simulink model "Bicycle_model_start"  (R2018a)
settings: Solver=VariableStepAuto  StartTime=0.0  StopTime=10.0  RelTol=1e-3
undefined symbols (not defined in the file): Ca, Cx, J, lf, lr, m, rwheel
libraries: simulink x1
settings Model: Creator=DvanHanswijk  LastModifiedBy=DvanHanswijk

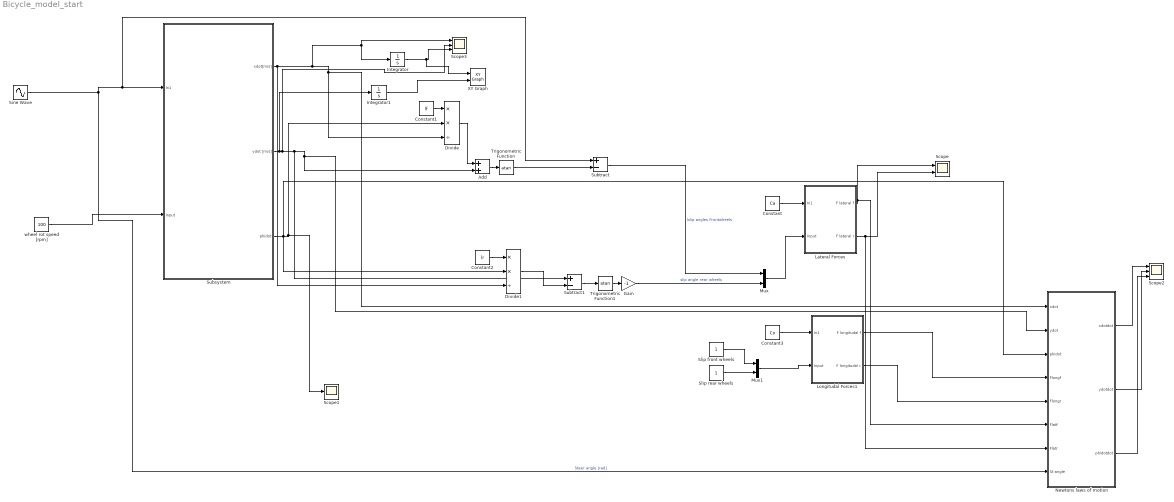
== system Bicycle_model_start ==
  Add : Sum
  Constant : Constant  Value=Ca
  Constant1 : Constant  Value=lf
  Constant2 : Constant  Value=lr
  Constant3 : Constant  Value=Cx
  Divide : Product  Inputs=**/
  Divide1 : Product  Inputs=**/
  Gain : Gain  Gain=-1
  Integrator : Integrator
  Integrator1 : Integrator
  Lateral Forces : Subsystem
  Longitudal Forces1 : Subsystem
  Mux : Mux  Inputs=2
  Mux1 : Mux  Inputs=2
  "Newtons laws of motion " : Subsystem
  Scope : Scope  NumInputPorts=2
  Scope1 : Scope
  Scope2 : Scope  NumInputPorts=3
  Scope3 : Scope  NumInputPorts=3
  Sine Wave : Sin  SampleTime=0
  "Slip front wheels " : Constant
  Slip rear wheels : Constant
  Subsystem : Subsystem
  Subtract : Sum  Inputs=+-
  Subtract1 : Sum  Inputs=+-
  Trigonometric Function : Trigonometry  Operator=atan
  Trigonometric Function1 : Trigonometry  Operator=atan
  XY Graph : simulink/Sinks/XY Graph  xmin=-1  xmax=10  ymin=-1  ymax=10  st=-1
  wheel rot speed [rpm] : Constant  Value=100
  wires:
  Constant/1 -> Lateral Forces/1(In1)
  Lateral Forces/1(F lateral f) -> "Newtons laws of motion "/6(Flatf), Scope/1
  Lateral Forces/2(F lateral r) -> "Newtons laws of motion "/7(Flatr), Scope/2
  wheel rot speed [rpm]/1 -> Subsystem/2(Input)
  Sine Wave/1 -> Subtract/1, Subsystem/1(In1), "Newtons laws of motion "/8(St angle)  "Steer angle [rad]"
  Mux/1 -> Lateral Forces/2(Input)
  Subtract/1 -> Mux/1  "lslip angles Frontwheels"
  Gain/1 -> Mux/2  "slip angle rear wheels"
  Trigonometric Function/1 -> Subtract/2
  Subsystem/2(ydot [m/s]) -> Integrator1/1, Scope3/2, Subtract1/1, "Newtons laws of motion "/2(ydot), Add/2
  Constant1/1 -> Divide/1
  Subsystem/3(phidot) -> "Newtons laws of motion "/3(phidot), Divide1/2, Scope1/1, Divide/2
  Subsystem/1(xdot[m/s]) -> Divide1/3, Integrator/1, Scope3/1, "Newtons laws of motion "/1(xdot), Divide/3
  Divide/1 -> Add/1
  Add/1 -> Trigonometric Function/1
  Trigonometric Function1/1 -> Gain/1
  Divide1/1 -> Subtract1/2
  Constant2/1 -> Divide1/1
  Subtract1/1 -> Trigonometric Function1/1
  Constant3/1 -> Longitudal Forces1/1(In1)
  "Slip front wheels "/1 -> Mux1/1
  Slip rear wheels/1 -> Mux1/2
  Mux1/1 -> Longitudal Forces1/2(Input)
  Longitudal Forces1/1(F longitudal f) -> "Newtons laws of motion "/4(Flongf)
  Longitudal Forces1/2(F longitudal r) -> "Newtons laws of motion "/5(Flongr)
  "Newtons laws of motion "/1(xdotdot) -> Scope2/1
  "Newtons laws of motion "/2(ydotdot) -> Scope2/2
  "Newtons laws of motion "/3(phidotdot) -> Scope2/3
  Integrator/1 -> XY Graph/1, Scope3/3
  Integrator1/1 -> XY Graph/2

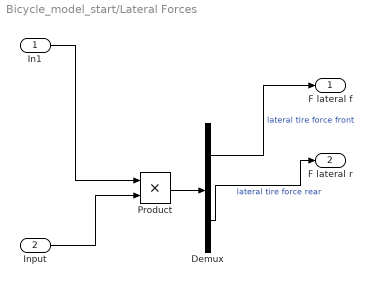
== system Bicycle_model_start/Lateral Forces ==
  In1 : Inport
  Input : Inport  Port=2
  Demux : Demux  Outputs=2
  Product : Product
  F lateral f : Outport
  F lateral r : Outport  Port=2
  wires:
  Input/1 -> Product/2
  Product/1 -> Demux/1
  Demux/2 -> F lateral r/1  "lateral tire force rear"
  Demux/1 -> F lateral f/1  "lateral tire force front"
  In1/1 -> Product/1

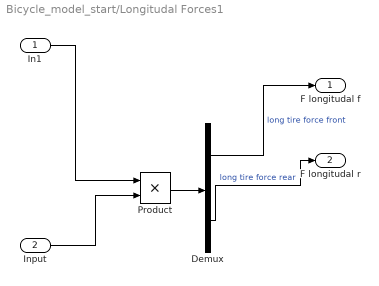
== system Bicycle_model_start/Longitudal Forces1 ==
  In1 : Inport
  Input : Inport  Port=2
  Demux : Demux  Outputs=2
  Product : Product
  F longitudal f : Outport
  F longitudal r : Outport  Port=2
  wires:
  In1/1 -> Product/1
  Demux/1 -> F longitudal f/1  "long tire force front"
  Demux/2 -> F longitudal r/1  "long tire force rear"
  Product/1 -> Demux/1
  Input/1 -> Product/2

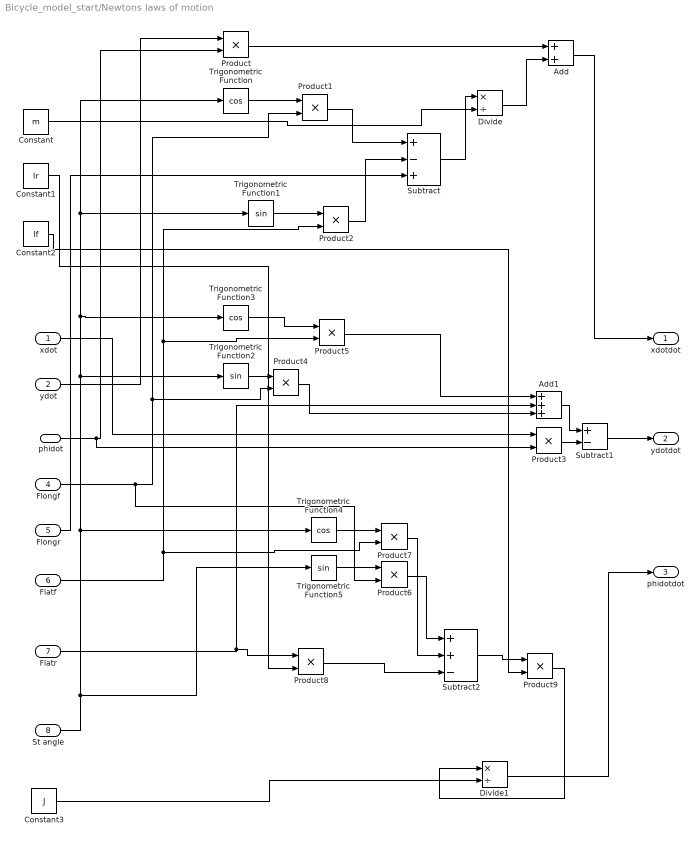
== system Bicycle_model_start/Newtons laws of motion  ==
  xdot : Inport
  ydot : Inport  Port=2
  phidot : Inport  Port=3
  Flongf : Inport  Port=4
  Flongr : Inport  Port=5
  Flatf : Inport  Port=6
  Flatr : Inport  Port=7
  St angle : Inport  Port=8
  Add : Sum
  Add1 : Sum  Inputs=3
  Constant : Constant  Value=m
  Constant1 : Constant  Value=lr
  Constant2 : Constant  Value=lf
  Constant3 : Constant  Value=J
  Divide : Product  Inputs=*/
  Divide1 : Product  Inputs=*/
  Product{,1..9} (10 alike) : Product
  Subtract : Sum  Inputs=+-+
  Subtract1 : Sum  Inputs=+-
  Subtract2 : Sum  Inputs=++-
  Trigonometric Function : Trigonometry  Operator=cos
  Trigonometric Function1 : Trigonometry
  Trigonometric Function2 : Trigonometry
  Trigonometric Function3 : Trigonometry  Operator=cos
  Trigonometric Function4 : Trigonometry  Operator=cos
  Trigonometric Function5 : Trigonometry
  xdotdot : Outport
  ydotdot : Outport  Port=2
  phidotdot : Outport  Port=3
  wires:
  ydot/1 -> Product/1
  phidot/1 -> Product3/2, Product/2
  St angle/1 -> Trigonometric Function5/1, Trigonometric Function4/1, Trigonometric Function3/1, Trigonometric Function1/1, Trigonometric Function/1, Trigonometric Function2/1
  Trigonometric Function/1 -> Product1/1
  Product1/1 -> Subtract/1
  Flatf/1 -> Product7/2, Product5/2, Product2/2
  Trigonometric Function1/1 -> Product2/1
  Product2/1 -> Subtract/2
  Flongr/1 -> Subtract/3
  Subtract/1 -> Divide/1
  Constant/1 -> Divide/2
  Product/1 -> Add/1
  Add/1 -> xdotdot/1
  Divide/1 -> Add/2
  Flongf/1 -> Product6/2, Product4/2, Product1/2
  Subtract1/1 -> ydotdot/1
  xdot/1 -> Product3/1
  Product3/1 -> Subtract1/2
  Trigonometric Function2/1 -> Product4/1
  Product4/1 -> Add1/3
  Add1/1 -> Subtract1/1
  Trigonometric Function3/1 -> Product5/1
  Flatr/1 -> Product8/1, Add1/2
  Product5/1 -> Add1/1
  Constant3/1 -> Divide1/2
  Trigonometric Function4/1 -> Product7/1
  Trigonometric Function5/1 -> Product6/1
  Constant1/1 -> Product8/2
  Product8/1 -> Subtract2/3
  Product6/1 -> Subtract2/1
  Product7/1 -> Subtract2/2
  Subtract2/1 -> Product9/1
  Constant2/1 -> Product9/2
  Product9/1 -> Divide1/1
  Divide1/1 -> phidotdot/1

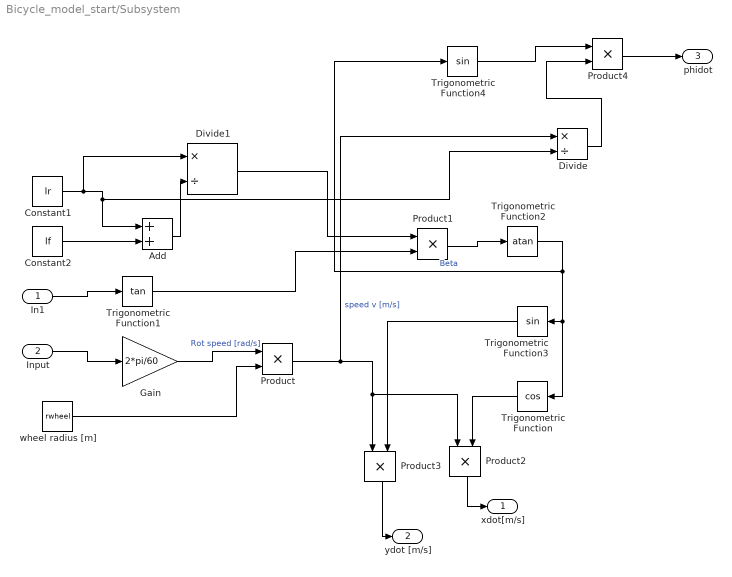
== system Bicycle_model_start/Subsystem ==
  In1 : Inport
  Input : Inport  Port=2
  Add : Sum
  Constant1 : Constant  Value=lr
  Constant2 : Constant  Value=lf
  Divide : Product  Inputs=*/
  Divide1 : Product  Inputs=*/
  Gain : Gain  Gain=2*pi/60
  Product{,1..4} (5 alike) : Product
  Trigonometric Function : Trigonometry  Operator=cos
  Trigonometric Function1 : Trigonometry  Operator=tan
  Trigonometric Function2 : Trigonometry  Operator=atan
  Trigonometric Function3 : Trigonometry
  Trigonometric Function4 : Trigonometry
  wheel radius [m] : Constant  Value=rwheel
  xdot[m/s] : Outport
  ydot [m/s] : Outport  Port=2
  phidot : Outport  Port=3
  wires:
  In1/1 -> Trigonometric Function1/1
  Trigonometric Function2/1 -> Trigonometric Function4/1, Trigonometric Function/1, Trigonometric Function3/1  "Beta"
  Gain/1 -> Product/1  "Rot speed [rad/s]"
  Product/1 -> Divide/1, Product2/1, Product3/1  "speed v [m/s]"
  wheel radius [m]/1 -> Product/2
  Add/1 -> Divide1/2
  Product1/1 -> Trigonometric Function2/1
  Divide1/1 -> Product1/1
  Constant2/1 -> Add/2
  Constant1/1 -> Divide1/1, Divide/2, Add/1
  Trigonometric Function1/1 -> Product1/2
  Input/1 -> Gain/1
  Trigonometric Function3/1 -> Product3/2
  Trigonometric Function/1 -> Product2/2
  Product2/1 -> xdot[m/s]/1
  Product3/1 -> ydot [m/s]/1
  Trigonometric Function4/1 -> Product4/1
  Divide/1 -> Product4/2
  Product4/1 -> phidot/1
